simulink model "LongDendriteCells"  (Simulink 7.1)
settings: Solver=ode45  StartTime=0.0  StopTime=1.5  RelTol=1e-3
libraries: NeuroModelerLibrary x61
settings Model: Creator=Bakhshiev  LastModifiedBy=Timba

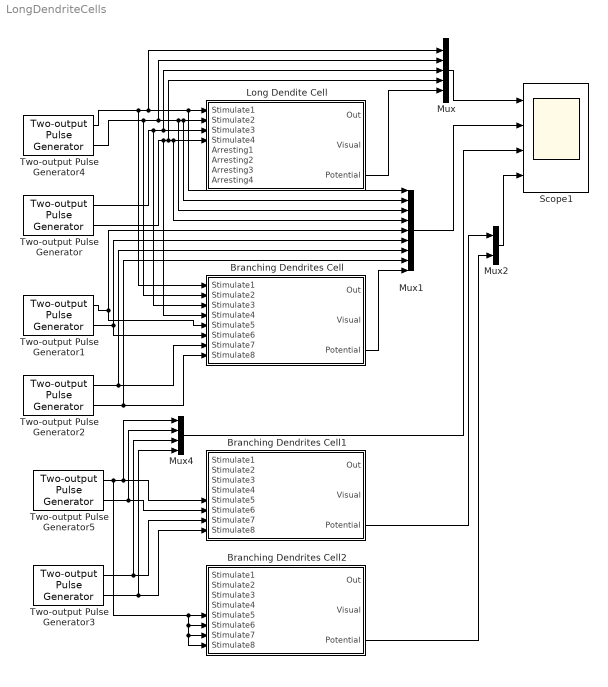
== system LongDendriteCells ==
  Branching Dendrites Cell : Subsystem  AncestorBlock=NeuroModelerLibrary/Dendrites Cells/Branching Dendrites Cell
  Branching Dendrites Cell1 : Subsystem  AncestorBlock=NeuroModelerLibrary/Dendrites Cells/Branching Dendrites Cell
  Branching Dendrites Cell2 : Subsystem  AncestorBlock=NeuroModelerLibrary/Dendrites Cells/Branching Dendrites Cell
  Long Dendite Cell : Subsystem  AncestorBlock=NeuroModelerLibrary/Dendrites Cells/Long Dendite Cell
  Mux : Mux  Inputs=5
  Mux1 : Mux  Inputs=9
  Mux2 : Mux  Inputs=2
  Mux4 : Mux
  Scope1 : Scope  NumInputPorts=4
      settings: YMin=0~0~0~0  YMax=1~1~1~0.075  MaxDataPoints=5000000
  Two-output Pulse Generator : NeuroModelerLibrary/Support/Two-output Pulse Generator  SystemSampleTime=-1  A=1  P1=200  P2=200  PW=1  ST=0.001  OOn1=0.9  OOff1=1.0  OOn2=1.1  OOff2=1.2
  Two-output Pulse Generator1 : NeuroModelerLibrary/Support/Two-output Pulse Generator  SystemSampleTime=-1  A=1  P1=200  P2=200  PW=1  ST=0.001  OOn1=0.55  OOff1=0.6  OOn2=0.72  OOff2=0.8
  Two-output Pulse Generator2 : NeuroModelerLibrary/Support/Two-output Pulse Generator  SystemSampleTime=-1  A=1  P1=200  P2=200  PW=1  ST=0.001  OOn1=0.95  OOff1=1.1  OOn2=1.12  OOff2=1.2
  Two-output Pulse Generator3 : NeuroModelerLibrary/Support/Two-output Pulse Generator  SystemSampleTime=-1  A=1  P1=200  P2=200  PW=1  ST=0.001  OOn1=0.6  OOff1=0.7  OOn2=0.65  OOff2=0.7
  Two-output Pulse Generator4 : NeuroModelerLibrary/Support/Two-output Pulse Generator  SystemSampleTime=-1  A=1  P1=200  P2=200  PW=1  ST=0.001  OOn1=0.5  OOff1=0.6  OOn2=0.7  OOff2=0.8
  Two-output Pulse Generator5 : NeuroModelerLibrary/Support/Two-output Pulse Generator  SystemSampleTime=-1  A=1  P1=200  P2=200  PW=1  ST=0.001  OOn1=0.5  OOff1=0.6  OOn2=0.55  OOff2=0.6
  wires:
  Two-output Pulse Generator4/1 -> Mux/1, Long Dendite Cell/1(Stimulate1), Mux1/1, Branching Dendrites Cell/1(Stimulate1)
  Two-output Pulse Generator4/2 -> Mux/2, Long Dendite Cell/2(Stimulate2), Mux1/2, Mux1/3, Branching Dendrites Cell/2(Stimulate2)
  Mux/1 -> Scope1/1
  Two-output Pulse Generator/2 -> Mux/4, Long Dendite Cell/4(Stimulate4), Mux1/4, Branching Dendrites Cell/4(Stimulate4)
  Two-output Pulse Generator/1 -> Mux/3, Long Dendite Cell/3(Stimulate3), Branching Dendrites Cell/3(Stimulate3)
  Long Dendite Cell/3(Potential) -> Mux/5
  Two-output Pulse Generator1/1 -> Branching Dendrites Cell/5(Stimulate5), Mux1/5
  Two-output Pulse Generator1/2 -> Branching Dendrites Cell/6(Stimulate6), Mux1/6
  Two-output Pulse Generator2/1 -> Branching Dendrites Cell/7(Stimulate7), Mux1/7
  Two-output Pulse Generator2/2 -> Branching Dendrites Cell/8(Stimulate8), Mux1/8
  Two-output Pulse Generator5/1 -> Branching Dendrites Cell1/5(Stimulate5), Mux4/1, Branching Dendrites Cell2/5(Stimulate5), Branching Dendrites Cell2/6(Stimulate6), Branching Dendrites Cell2/7(Stimulate7), Branching Dendrites Cell2/8(Stimulate8)
  Two-output Pulse Generator5/2 -> Branching Dendrites Cell1/6(Stimulate6), Mux4/2
  Two-output Pulse Generator3/1 -> Branching Dendrites Cell1/7(Stimulate7), Mux4/3
  Two-output Pulse Generator3/2 -> Branching Dendrites Cell1/8(Stimulate8), Mux4/4
  Mux2/1 -> Scope1/4
  Branching Dendrites Cell2/3(Potential) -> Mux2/2
  Branching Dendrites Cell1/3(Potential) -> Mux2/1
  Mux4/1 -> Scope1/3
  Branching Dendrites Cell/3(Potential) -> Mux1/9
  Mux1/1 -> Scope1/2

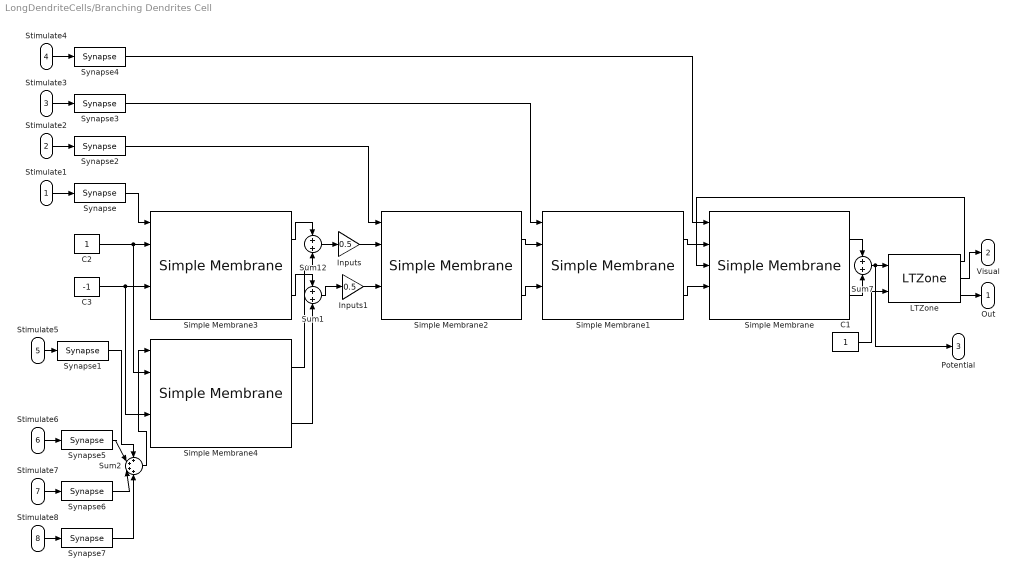
== system LongDendriteCells/Branching Dendrites Cell ==
  Stimulate1 : Inport  OutDataType=sfix(16)  OutScaling=2^0
  Stimulate2 : Inport  Port=2  OutDataType=sfix(16)  OutScaling=2^0
  Stimulate3 : Inport  Port=3  OutDataType=sfix(16)  OutScaling=2^0
  Stimulate4 : Inport  Port=4  OutDataType=sfix(16)  OutScaling=2^0
  Stimulate5 : Inport  Port=5  OutDataType=sfix(16)  OutScaling=2^0
  Stimulate6 : Inport  Port=6  OutDataType=sfix(16)  OutScaling=2^0
  Stimulate7 : Inport  Port=7  OutDataType=sfix(16)  OutScaling=2^0
  Stimulate8 : Inport  Port=8  OutDataType=sfix(16)  OutScaling=2^0
  C1 : Constant  OutDataType=sfix(16)  OutScaling=2^0
  C2 : Constant  OutDataType=sfix(16)  OutScaling=2^0
  C3 : Constant  Value=-1  OutDataType=sfix(16)  OutScaling=2^0
  Inputs : Gain  Gain=0.5  ParameterDataType=sfix(16)  ParameterScaling=2^0  OutDataType=sfix(16)  OutScaling=2^0  OutDataTypeStr=Inherit: Same as input  ParamDataTypeStr=Inherit: Same as input
  Inputs1 : Gain  Gain=0.5  ParameterDataType=sfix(16)  ParameterScaling=2^0  OutDataType=sfix(16)  OutScaling=2^0  OutDataTypeStr=Inherit: Same as input  ParamDataTypeStr=Inherit: Same as input
  LTZone : NeuroModelerLibrary/Neuron Elements/LTZone  SystemSampleTime=-1  NM=1  FB=2  IT=0.005  T=0.1
  Simple Membrane{,1..4} (5 alike) : NeuroModelerLibrary/Neuron Elements/Simple Membrane  SystemSampleTime=-1  ACm=1e-9  ARm=1e7  ECm=1e-9  ERm=1e7  ARFm=1e8  ERFm=1e8
  Sum1 : Sum  OutDataType=sfix(16)  OutScaling=2^0  SaturateOnIntegerOverflow=on  InputSameDT=on  OutDataTypeStr=Inherit: Same as first input
  Sum12 : Sum  OutDataType=sfix(16)  OutScaling=2^0  SaturateOnIntegerOverflow=on  InputSameDT=on  OutDataTypeStr=Inherit: Same as first input
  Sum2 : Sum  Inputs=++++  OutDataType=sfix(16)  OutScaling=2^0  SaturateOnIntegerOverflow=on  InputSameDT=on  OutDataTypeStr=Inherit: Same as first input
  Sum7 : Sum  OutDataType=sfix(16)  OutScaling=2^0  SaturateOnIntegerOverflow=on  InputSameDT=on  OutDataTypeStr=Inherit: Same as first input
  Synapse{,1..7} (8 alike) : NeuroModelerLibrary/Neuron Elements/Synapse  SystemSampleTime=-1  SecretionTC=0.001  DecompositionTC=0.01  ksi=1  gamma=1e8
  Out : Outport  OutDataType=sfix(16)  OutScaling=2^0
  Visual : Outport  Port=2  OutDataType=sfix(16)  OutScaling=2^0
  Potential : Outport  Port=3  OutDataType=sfix(16)  OutScaling=2^0
  wires:
  Synapse5/1 -> Sum2/2
  Inputs1/1 -> Simple Membrane2/4
  Inputs/1 -> Simple Membrane2/2
  Synapse1/1 -> Sum2/1
  Sum2/1 -> Simple Membrane4/1
  Simple Membrane2/2 -> Simple Membrane1/4
  Simple Membrane2/1 -> Simple Membrane1/2
  Simple Membrane3/1 -> Sum12/1
  Simple Membrane3/2 -> Sum1/1
  Sum1/1 -> Inputs1/1
  Sum12/1 -> Inputs/1
  Simple Membrane4/1 -> Sum12/2
  Simple Membrane4/2 -> Sum1/2
  Simple Membrane/2 -> Sum7/2
  Simple Membrane/1 -> Sum7/1
  LTZone/1 -> Simple Membrane/3
  Sum7/1 -> LTZone/1, Potential/1
  Simple Membrane1/2 -> Simple Membrane/4
  Simple Membrane1/1 -> Simple Membrane/2
  Stimulate5/1 -> Synapse1/1
  Stimulate1/1 -> Synapse/1
  C1/1 -> LTZone/2
  LTZone/3 -> Out/1
  LTZone/2 -> Visual/1
  C3/1 -> Simple Membrane3/4, Simple Membrane4/4
  C2/1 -> Simple Membrane3/2, Simple Membrane4/2
  Synapse/1 -> Simple Membrane3/1
  Synapse2/1 -> Simple Membrane2/1
  Stimulate2/1 -> Synapse2/1
  Synapse3/1 -> Simple Membrane1/1
  Stimulate3/1 -> Synapse3/1
  Synapse4/1 -> Simple Membrane/1
  Stimulate4/1 -> Synapse4/1
  Stimulate6/1 -> Synapse5/1
  Stimulate7/1 -> Synapse6/1
  Synapse6/1 -> Sum2/3
  Stimulate8/1 -> Synapse7/1
  Synapse7/1 -> Sum2/4

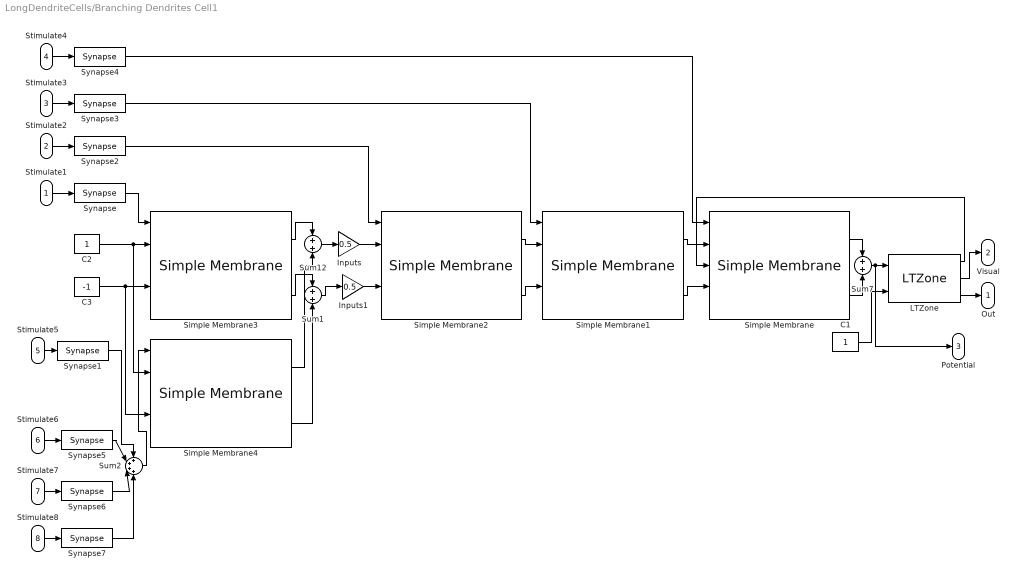
== system LongDendriteCells/Branching Dendrites Cell1 ==
  Stimulate1 : Inport  OutDataType=sfix(16)  OutScaling=2^0
  Stimulate2 : Inport  Port=2  OutDataType=sfix(16)  OutScaling=2^0
  Stimulate3 : Inport  Port=3  OutDataType=sfix(16)  OutScaling=2^0
  Stimulate4 : Inport  Port=4  OutDataType=sfix(16)  OutScaling=2^0
  Stimulate5 : Inport  Port=5  OutDataType=sfix(16)  OutScaling=2^0
  Stimulate6 : Inport  Port=6  OutDataType=sfix(16)  OutScaling=2^0
  Stimulate7 : Inport  Port=7  OutDataType=sfix(16)  OutScaling=2^0
  Stimulate8 : Inport  Port=8  OutDataType=sfix(16)  OutScaling=2^0
  C1 : Constant  OutDataType=sfix(16)  OutScaling=2^0
  C2 : Constant  OutDataType=sfix(16)  OutScaling=2^0
  C3 : Constant  Value=-1  OutDataType=sfix(16)  OutScaling=2^0
  Inputs : Gain  Gain=0.5  ParameterDataType=sfix(16)  ParameterScaling=2^0  OutDataType=sfix(16)  OutScaling=2^0  OutDataTypeStr=Inherit: Same as input  ParamDataTypeStr=Inherit: Same as input
  Inputs1 : Gain  Gain=0.5  ParameterDataType=sfix(16)  ParameterScaling=2^0  OutDataType=sfix(16)  OutScaling=2^0  OutDataTypeStr=Inherit: Same as input  ParamDataTypeStr=Inherit: Same as input
  LTZone : NeuroModelerLibrary/Neuron Elements/LTZone  SystemSampleTime=-1  NM=1  FB=2  IT=0.005  T=0.1
  Simple Membrane{,1..4} (5 alike) : NeuroModelerLibrary/Neuron Elements/Simple Membrane  SystemSampleTime=-1  ACm=1e-9  ARm=1e7  ECm=1e-9  ERm=1e7  ARFm=1e8  ERFm=1e8
  Sum1 : Sum  OutDataType=sfix(16)  OutScaling=2^0  SaturateOnIntegerOverflow=on  InputSameDT=on  OutDataTypeStr=Inherit: Same as first input
  Sum12 : Sum  OutDataType=sfix(16)  OutScaling=2^0  SaturateOnIntegerOverflow=on  InputSameDT=on  OutDataTypeStr=Inherit: Same as first input
  Sum2 : Sum  Inputs=++++  OutDataType=sfix(16)  OutScaling=2^0  SaturateOnIntegerOverflow=on  InputSameDT=on  OutDataTypeStr=Inherit: Same as first input
  Sum7 : Sum  OutDataType=sfix(16)  OutScaling=2^0  SaturateOnIntegerOverflow=on  InputSameDT=on  OutDataTypeStr=Inherit: Same as first input
  Synapse{,1..7} (8 alike) : NeuroModelerLibrary/Neuron Elements/Synapse  SystemSampleTime=-1  SecretionTC=0.001  DecompositionTC=0.01  ksi=1  gamma=1e8
  Out : Outport  OutDataType=sfix(16)  OutScaling=2^0
  Visual : Outport  Port=2  OutDataType=sfix(16)  OutScaling=2^0
  Potential : Outport  Port=3  OutDataType=sfix(16)  OutScaling=2^0
  wires:
  Synapse5/1 -> Sum2/2
  Inputs1/1 -> Simple Membrane2/4
  Inputs/1 -> Simple Membrane2/2
  Synapse1/1 -> Sum2/1
  Sum2/1 -> Simple Membrane4/1
  Simple Membrane2/2 -> Simple Membrane1/4
  Simple Membrane2/1 -> Simple Membrane1/2
  Simple Membrane3/1 -> Sum12/1
  Simple Membrane3/2 -> Sum1/1
  Sum1/1 -> Inputs1/1
  Sum12/1 -> Inputs/1
  Simple Membrane4/1 -> Sum12/2
  Simple Membrane4/2 -> Sum1/2
  Simple Membrane/2 -> Sum7/2
  Simple Membrane/1 -> Sum7/1
  LTZone/1 -> Simple Membrane/3
  Sum7/1 -> LTZone/1, Potential/1
  Simple Membrane1/2 -> Simple Membrane/4
  Simple Membrane1/1 -> Simple Membrane/2
  Stimulate5/1 -> Synapse1/1
  Stimulate1/1 -> Synapse/1
  C1/1 -> LTZone/2
  LTZone/3 -> Out/1
  LTZone/2 -> Visual/1
  C3/1 -> Simple Membrane3/4, Simple Membrane4/4
  C2/1 -> Simple Membrane3/2, Simple Membrane4/2
  Synapse/1 -> Simple Membrane3/1
  Synapse2/1 -> Simple Membrane2/1
  Stimulate2/1 -> Synapse2/1
  Synapse3/1 -> Simple Membrane1/1
  Stimulate3/1 -> Synapse3/1
  Synapse4/1 -> Simple Membrane/1
  Stimulate4/1 -> Synapse4/1
  Stimulate6/1 -> Synapse5/1
  Stimulate7/1 -> Synapse6/1
  Synapse6/1 -> Sum2/3
  Stimulate8/1 -> Synapse7/1
  Synapse7/1 -> Sum2/4

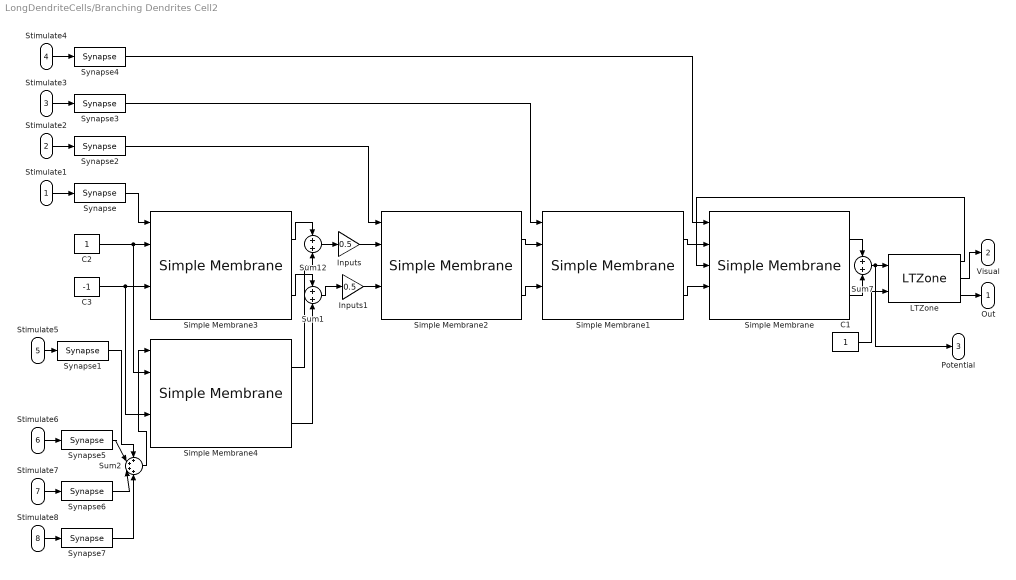
== system LongDendriteCells/Branching Dendrites Cell2 ==
  Stimulate1 : Inport  OutDataType=sfix(16)  OutScaling=2^0
  Stimulate2 : Inport  Port=2  OutDataType=sfix(16)  OutScaling=2^0
  Stimulate3 : Inport  Port=3  OutDataType=sfix(16)  OutScaling=2^0
  Stimulate4 : Inport  Port=4  OutDataType=sfix(16)  OutScaling=2^0
  Stimulate5 : Inport  Port=5  OutDataType=sfix(16)  OutScaling=2^0
  Stimulate6 : Inport  Port=6  OutDataType=sfix(16)  OutScaling=2^0
  Stimulate7 : Inport  Port=7  OutDataType=sfix(16)  OutScaling=2^0
  Stimulate8 : Inport  Port=8  OutDataType=sfix(16)  OutScaling=2^0
  C1 : Constant  OutDataType=sfix(16)  OutScaling=2^0
  C2 : Constant  OutDataType=sfix(16)  OutScaling=2^0
  C3 : Constant  Value=-1  OutDataType=sfix(16)  OutScaling=2^0
  Inputs : Gain  Gain=0.5  ParameterDataType=sfix(16)  ParameterScaling=2^0  OutDataType=sfix(16)  OutScaling=2^0  OutDataTypeStr=Inherit: Same as input  ParamDataTypeStr=Inherit: Same as input
  Inputs1 : Gain  Gain=0.5  ParameterDataType=sfix(16)  ParameterScaling=2^0  OutDataType=sfix(16)  OutScaling=2^0  OutDataTypeStr=Inherit: Same as input  ParamDataTypeStr=Inherit: Same as input
  LTZone : NeuroModelerLibrary/Neuron Elements/LTZone  SystemSampleTime=-1  NM=1  FB=2  IT=0.005  T=0.1
  Simple Membrane{,1..4} (5 alike) : NeuroModelerLibrary/Neuron Elements/Simple Membrane  SystemSampleTime=-1  ACm=1e-9  ARm=1e7  ECm=1e-9  ERm=1e7  ARFm=1e8  ERFm=1e8
  Sum1 : Sum  OutDataType=sfix(16)  OutScaling=2^0  SaturateOnIntegerOverflow=on  InputSameDT=on  OutDataTypeStr=Inherit: Same as first input
  Sum12 : Sum  OutDataType=sfix(16)  OutScaling=2^0  SaturateOnIntegerOverflow=on  InputSameDT=on  OutDataTypeStr=Inherit: Same as first input
  Sum2 : Sum  Inputs=++++  OutDataType=sfix(16)  OutScaling=2^0  SaturateOnIntegerOverflow=on  InputSameDT=on  OutDataTypeStr=Inherit: Same as first input
  Sum7 : Sum  OutDataType=sfix(16)  OutScaling=2^0  SaturateOnIntegerOverflow=on  InputSameDT=on  OutDataTypeStr=Inherit: Same as first input
  Synapse{,1..7} (8 alike) : NeuroModelerLibrary/Neuron Elements/Synapse  SystemSampleTime=-1  SecretionTC=0.001  DecompositionTC=0.01  ksi=1  gamma=1e8
  Out : Outport  OutDataType=sfix(16)  OutScaling=2^0
  Visual : Outport  Port=2  OutDataType=sfix(16)  OutScaling=2^0
  Potential : Outport  Port=3  OutDataType=sfix(16)  OutScaling=2^0
  wires:
  Synapse5/1 -> Sum2/2
  Inputs1/1 -> Simple Membrane2/4
  Inputs/1 -> Simple Membrane2/2
  Synapse1/1 -> Sum2/1
  Sum2/1 -> Simple Membrane4/1
  Simple Membrane2/2 -> Simple Membrane1/4
  Simple Membrane2/1 -> Simple Membrane1/2
  Simple Membrane3/1 -> Sum12/1
  Simple Membrane3/2 -> Sum1/1
  Sum1/1 -> Inputs1/1
  Sum12/1 -> Inputs/1
  Simple Membrane4/1 -> Sum12/2
  Simple Membrane4/2 -> Sum1/2
  Simple Membrane/2 -> Sum7/2
  Simple Membrane/1 -> Sum7/1
  LTZone/1 -> Simple Membrane/3
  Sum7/1 -> LTZone/1, Potential/1
  Simple Membrane1/2 -> Simple Membrane/4
  Simple Membrane1/1 -> Simple Membrane/2
  Stimulate5/1 -> Synapse1/1
  Stimulate1/1 -> Synapse/1
  C1/1 -> LTZone/2
  LTZone/3 -> Out/1
  LTZone/2 -> Visual/1
  C3/1 -> Simple Membrane3/4, Simple Membrane4/4
  C2/1 -> Simple Membrane3/2, Simple Membrane4/2
  Synapse/1 -> Simple Membrane3/1
  Synapse2/1 -> Simple Membrane2/1
  Stimulate2/1 -> Synapse2/1
  Synapse3/1 -> Simple Membrane1/1
  Stimulate3/1 -> Synapse3/1
  Synapse4/1 -> Simple Membrane/1
  Stimulate4/1 -> Synapse4/1
  Stimulate6/1 -> Synapse5/1
  Stimulate7/1 -> Synapse6/1
  Synapse6/1 -> Sum2/3
  Stimulate8/1 -> Synapse7/1
  Synapse7/1 -> Sum2/4

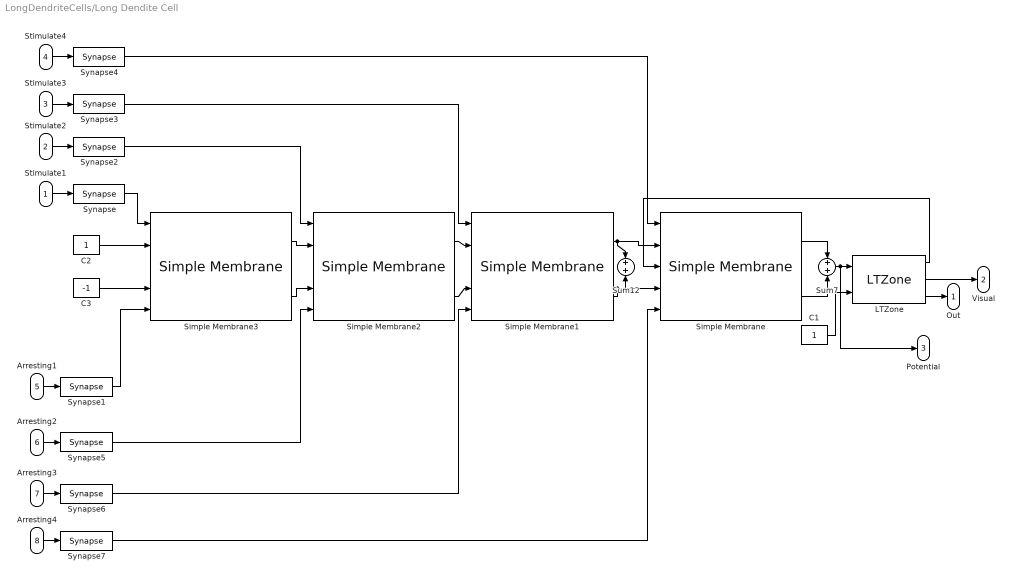
== system LongDendriteCells/Long Dendite Cell ==
  Stimulate1 : Inport  OutDataType=sfix(16)  OutScaling=2^0
  Stimulate2 : Inport  Port=2  OutDataType=sfix(16)  OutScaling=2^0
  Stimulate3 : Inport  Port=3  OutDataType=sfix(16)  OutScaling=2^0
  Stimulate4 : Inport  Port=4  OutDataType=sfix(16)  OutScaling=2^0
  Arresting1 : Inport  Port=5  OutDataType=sfix(16)  OutScaling=2^0
  Arresting2 : Inport  Port=6  OutDataType=sfix(16)  OutScaling=2^0
  Arresting3 : Inport  Port=7  OutDataType=sfix(16)  OutScaling=2^0
  Arresting4 : Inport  Port=8  OutDataType=sfix(16)  OutScaling=2^0
  C1 : Constant  OutDataType=sfix(16)  OutScaling=2^0
  C2 : Constant  OutDataType=sfix(16)  OutScaling=2^0
  C3 : Constant  Value=-1  OutDataType=sfix(16)  OutScaling=2^0
  LTZone : NeuroModelerLibrary/Neuron Elements/LTZone  SystemSampleTime=-1  NM=1  FB=2  IT=0.005  T=0.1
  Simple Membrane{,1..3} (4 alike) : NeuroModelerLibrary/Neuron Elements/Simple Membrane  SystemSampleTime=-1  ACm=1e-9  ARm=1e7  ECm=1e-9  ERm=1e7  ARFm=1e8  ERFm=1e8
  Sum12 : Sum  OutDataType=sfix(16)  OutScaling=2^0  SaturateOnIntegerOverflow=on  InputSameDT=on  OutDataTypeStr=Inherit: Same as first input
  Sum7 : Sum  OutDataType=sfix(16)  OutScaling=2^0  SaturateOnIntegerOverflow=on  InputSameDT=on  OutDataTypeStr=Inherit: Same as first input
  Synapse{,1..7} (8 alike) : NeuroModelerLibrary/Neuron Elements/Synapse  SystemSampleTime=-1  SecretionTC=0.001  DecompositionTC=0.01  ksi=1  gamma=1e8
  Out : Outport  OutDataType=sfix(16)  OutScaling=2^0
  Visual : Outport  Port=2  OutDataType=sfix(16)  OutScaling=2^0
  Potential : Outport  Port=3  OutDataType=sfix(16)  OutScaling=2^0
  wires:
  Synapse7/1 -> Simple Membrane/5
  Arresting4/1 -> Synapse7/1
  Synapse6/1 -> Simple Membrane1/5
  Arresting3/1 -> Synapse6/1
  Synapse5/1 -> Simple Membrane2/5
  Arresting2/1 -> Synapse5/1
  Stimulate4/1 -> Synapse4/1
  Synapse4/1 -> Simple Membrane/1
  Stimulate3/1 -> Synapse3/1
  Synapse3/1 -> Simple Membrane1/1
  Stimulate2/1 -> Synapse2/1
  Synapse2/1 -> Simple Membrane2/1
  Synapse/1 -> Simple Membrane3/1
  C2/1 -> Simple Membrane3/2
  C3/1 -> Simple Membrane3/4
  Synapse1/1 -> Simple Membrane3/5
  Simple Membrane3/2 -> Simple Membrane2/4
  Simple Membrane3/1 -> Simple Membrane2/2
  Simple Membrane2/2 -> Simple Membrane1/4
  Simple Membrane2/1 -> Simple Membrane1/2
  LTZone/2 -> Visual/1
  LTZone/3 -> Out/1
  C1/1 -> LTZone/2
  Stimulate1/1 -> Synapse/1
  Arresting1/1 -> Synapse1/1
  Simple Membrane1/1 -> Simple Membrane/2, Sum12/1
  Simple Membrane1/2 -> Simple Membrane/4, Sum12/2
  Sum7/1 -> LTZone/1, Potential/1
  LTZone/1 -> Simple Membrane/3
  Simple Membrane/1 -> Sum7/1
  Simple Membrane/2 -> Sum7/2
